simulink model "compensator_lag"  (R2022b)
settings: Solver=VariableStepAuto  StartTime=0.0  StopTime=10.0  RelTol=1e-3
libraries: simulink_extras x5
settings Model: Creator=integzz  LastModifiedBy=integzz

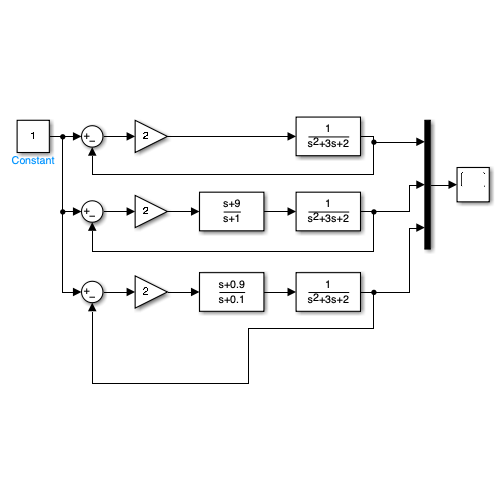
[thumbnail: Simulink's stored preview of the top-level diagram]
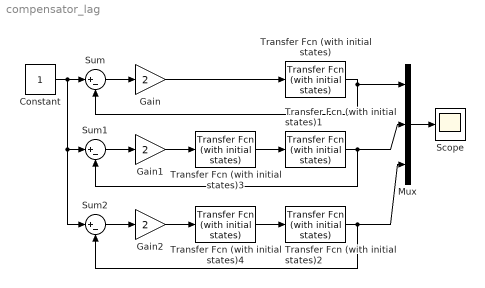
== system compensator_lag ==
  Constant : Constant
  Gain : Gain  Gain=2
  Gain1 : Gain  Gain=2
  Gain2 : Gain  Gain=2
  Mux : Mux  Inputs=3
  Scope : Scope
  Sum : Sum  Inputs=|+-
  Sum1 : Sum  Inputs=|+-
  Sum2 : Sum  Inputs=|+-
  Transfer Fcn (with initial states) : simulink_extras/Additional Linear/Transfer Fcn (with initial states)  N=[1]  D=[1 3 2]  X0=0
  Transfer Fcn (with initial states)1 : simulink_extras/Additional Linear/Transfer Fcn (with initial states)  N=[1]  D=[1 3 2]  X0=0
  Transfer Fcn (with initial states)2 : simulink_extras/Additional Linear/Transfer Fcn (with initial states)  N=[1]  D=[1 3 2]  X0=0
  Transfer Fcn (with initial states)3 : simulink_extras/Additional Linear/Transfer Fcn (with initial states)  N=[1 9]  D=[1 1]  X0=0
  Transfer Fcn (with initial states)4 : simulink_extras/Additional Linear/Transfer Fcn (with initial states)  N=[1 0.9]  D=[1 0.1]  X0=0
  wires:
  Gain/1 -> Transfer Fcn (with initial states)/1
  Sum/1 -> Gain/1
  Transfer Fcn (with initial states)/1 -> Sum/2, Mux/1
  Transfer Fcn (with initial states)1/1 -> Mux/2, Sum1/2
  Sum1/1 -> Gain1/1
  Gain1/1 -> Transfer Fcn (with initial states)3/1
  Gain2/1 -> Transfer Fcn (with initial states)4/1
  Constant/1 -> Sum2/1, Sum1/1, Sum/1
  Sum2/1 -> Gain2/1
  Transfer Fcn (with initial states)2/1 -> Sum2/2, Mux/3
  Mux/1 -> Scope/1
  Transfer Fcn (with initial states)3/1 -> Transfer Fcn (with initial states)1/1
  Transfer Fcn (with initial states)4/1 -> Transfer Fcn (with initial states)2/1
